simulink model "step_cmodel02_cl_2xPol"  (Simulink 7.9)
settings: Solver=ode45  StartTime=0.0  StopTime=10.0  RelTol=1e-3
values from neighbouring files (symbols this model uses):
  height = tool(1,3)-0.27    [2xPol.m]    (also in cmodel_data.m = 0.37)
  initE = -1    [2xPol.m]
  intrinsic = 779.280    (= 779.28)    [cmodel_data.m]
  radius = 0.579106    [2xPol.m]    (also in cmodel_data.m = 0.6)
  T = 0.01786    [cmodel_data.m]
undefined symbols (not defined in the file or in its folder): gain
settings Model: Creator=ex16  LastModifiedBy=ex16

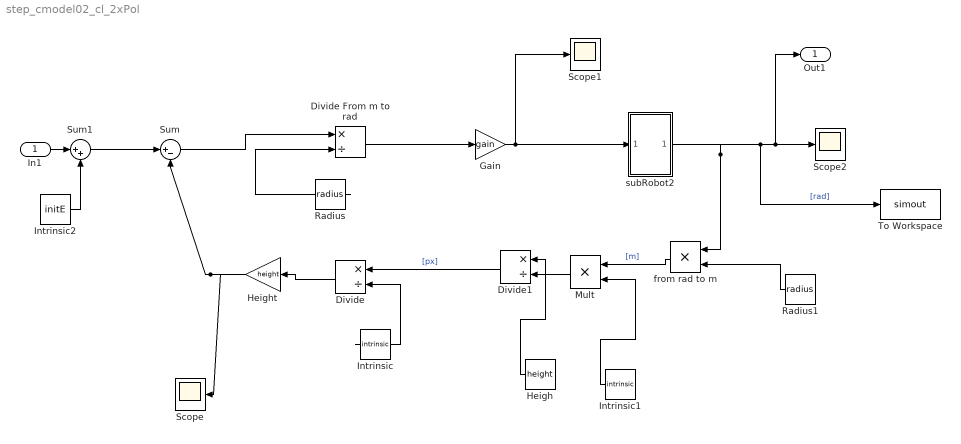
== system step_cmodel02_cl_2xPol ==
  In1 : Inport
  Divide : Product  Inputs=*/
  Divide From m to rad : Product  Inputs=*/
  Divide1 : Product  Inputs=*/
  Gain : Gain  Gain=gain
  Heigh : Constant  Value=height
  Height : Gain  Gain=height
  Intrinsic : Constant  Value=intrinsic
  Intrinsic1 : Constant  Value=intrinsic
  Intrinsic2 : Constant  Value=initE
  Mult : Product  Inputs=**
  Radius : Constant  Value=radius
  Radius1 : Constant  Value=radius
  Scope : Scope
  Scope1 : Scope
      settings: SaveName=ScopeData3
  Scope2 : Scope
      settings: SaveName=ScopeData4
  Sum : Sum  Inputs=|+-
  Sum1 : Sum  Inputs=|++
  To Workspace : ToWorkspace  VariableName=simout  SampleTime=-1  SaveFormat=Structure With Time
  from rad to m : Product  Inputs=**
  subRobot2 : Subsystem
  Out1 : Outport
  wires:
  Intrinsic/1 -> Divide/2
  Divide/1 -> Height/1
  Height/1 -> Scope/1, Sum/2
  Radius/1 -> Divide From m to rad/2
  subRobot2/1(Out1) -> from rad to m/1, To Workspace/1, Scope2/1, Out1/1  "[rad]"
  Radius1/1 -> from rad to m/2
  Heigh/1 -> Divide1/2
  Mult/1 -> Divide1/1
  Intrinsic1/1 -> Mult/2
  from rad to m/1 -> Mult/1  "[m]"
  Divide1/1 -> Divide/1  "[px]"
  Sum/1 -> Divide From m to rad/1
  Divide From m to rad/1 -> Gain/1
  Gain/1 -> Scope1/1, subRobot2/1(In1)
  Intrinsic2/1 -> Sum1/2
  In1/1 -> Sum1/1
  Sum1/1 -> Sum/1

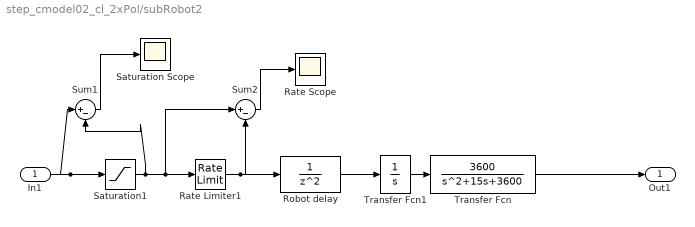
== system step_cmodel02_cl_2xPol/subRobot2 ==
  In1 : Inport
  Rate Limiter1 : RateLimiter  RisingSlewLimit=15  FallingSlewLimit=-15  SampleTimeMode=inherited
  Rate Scope : Scope
      settings: TimeRange=2  YMin=0  YMax=0.25  SaveName=ScopeData2
  Robot delay : DiscreteTransferFcn  Denominator=[1 0 0]  SampleTime=T
  Saturation Scope : Scope
  Saturation1 : Saturate  UpperLimit=3.2  LowerLimit=-3.2  SampleTime=T
  Sum1 : Sum  Inputs=|+-
  Sum2 : Sum  Inputs=|+-
  Transfer Fcn : TransferFcn  Numerator=[3600]  Denominator=[1 15 3600]
  Transfer Fcn1 : TransferFcn  Denominator=[1 0]
  Out1 : Outport
  wires:
  Saturation1/1 -> Rate Limiter1/1, Sum2/1, Sum1/2
  Rate Limiter1/1 -> Robot delay/1, Sum2/2
  Sum2/1 -> Rate Scope/1
  In1/1 -> Saturation1/1, Sum1/1
  Sum1/1 -> Saturation Scope/1
  Transfer Fcn1/1 -> Transfer Fcn/1
  Robot delay/1 -> Transfer Fcn1/1
  Transfer Fcn/1 -> Out1/1
